simulink library "dspsigops"  (Simulink 6.0)
settings: Solver=ode45  SolverMode=SingleTasking  StartTime=0.0  StopTime=10.0  RelTol=1e-3
values from neighbouring files (symbols this model uses):
  b = tmp(end-3:end)    [aboutdspblks.m]    (also in dspcsum.m = find_system(blk,'LookUnderMasks','all', 'FollowLinks','on', ; dspfdes.m = []; dsprprim.m = b+Li)
settings Model: RequirementInfo=9  CovMetricSettings=d  ForwardingTableString=||__slOldName__||dspsigops/Integer Delay||__slNewName__||dspobslib/Integer Delay  Creator=szlotkin  LastModifiedBy=mlongfri  ExtModeAutoUpdateStatusClock=off  ProdHWDeviceType=Specified
settings DataIOCC: SignalLoggingName=logsOut
settings OptimizationCC: BooleanDataType=off
settings DebuggingCC: CheckExecutionContextPreStartOutputMsg=on  CheckExecutionContextRuntimeOutputMsg=on  SolverPrmCheckMsg=none
settings HardwareCC: ProdHWDeviceType=Specified  TargetUnknown=on
settings ModelReferenceCC: UpdateModelReferenceTargets=IfOutOfDate
settings SFSimCC: SFSimApplyToAllLibs=on  SFSimBuildMode=Incremental

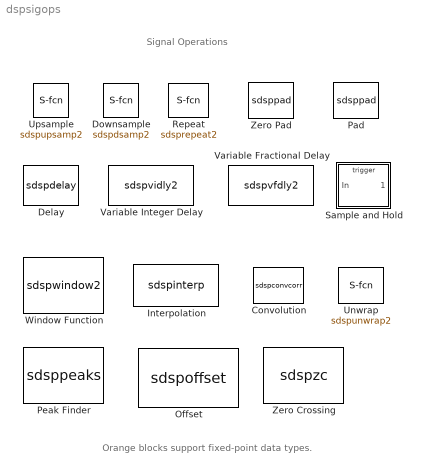
== system dspsigops ==
  note: Signal Operations
  note: Orange blocks support fixed-point data types.
  Convolution : S-Function  DialogController=dspDDGCreate  DialogControllerArgs=DataTag0  FunctionName=sdspconvcorr  Parameters=domain,0,dtInfo.prodOutputMode,dtInfo.prodOutputWordLength,dtInfo.prodOutputFracLength,dtInfo.accumMode,dtInfo.accumWordLength,dtInfo.accumFracLength,dtInfo.outputMode,dtInfo.outputWordLength,dtInfo.outputFracLength,dtInfo.roundingMode,dtInfo.overflowMode  mask(Convolution){domain=Time, additionalParams=off, allowOverrides=on, outputMode=Same as accumulator, outputWordLength=16, outputFracLength=15, accumMode=Inherit via internal rule, accumWordLength=32, accumFracLength=30, prodOutputMode=Inherit via internal rule, prodOutputWordLength=32, prodOutputFracLength=30, roundingMode=Floor, overflowMode=off, LockScale=off}
      mask prompts: domain "Computation domain:"; additionalParams "------- Show additional parameters -------"; allowOverrides "Allow overrides from DSP Fixed-Point Attributes blocks"; outputMode "Fixed-point output attributes:"; outputWordLength "Output word length:"; outputFracLength "Output fraction length:"; accumMode "Fixed-point accumulator attributes:"; accumWordLength "Accumulator word length:"; accumFracLength "Accumulator fraction length:"; prodOutputMode "Fixed-point product output attributes:"; prodOutputWordLength "Product output word length:"; prodOutputFracLength "Product output fraction length:"; roundingMode "Round integer calculations toward:"; overflowMode "Saturate on integer overflow"; LockScale "Lock scaling"
      mask help: Convolve two inputs. The block computes in the time domain or frequency domain. To minimize the number of computations, select "Fastest" in the Computation domain parameter. To minimize memory use, select "Time" in the Computation domain parameter.
      mask init:
      | dtInfo = dspblkconvcorr('init');
      settings: CopyFcn=dspfixptcopycallback
      mask Help: web(dspbhelp);
      mask StyleString: popup(Time|Frequency|Fastest),checkbox,checkbox,popup(Same as accumulator|Same as product output|Same as first input|Binary point scaling|Slope and bias scaling|User-defined),edit,edit,popup(Inherit via internal rule|Same as product output|Same as first input|Binary point scaling|Slope and bias scaling|User-defined),edit,edit,popup(Inherit via internal rule|Same as first input|Binary point scaling|Slope and bias scaling|User-defined),edit,edit,popup(Floor|Nearest),checkbox,checkbox
      mask Display: disp('CONV')
  Delay : S-Function  FunctionName=sdspdelay  Parameters=dly_unit, delay, ic_detail, dif_ic_for_ch, dif_ic_for_dly, ic, reset  mask(Delay){dly_unit=Sample, delay=1, ic_detail=off, dif_ic_for_ch=off, dif_ic_for_dly=off, ic=0, reset_popup=None}
      mask prompts: dly_unit "Delay units:"; delay "Delay (samples):"; ic_detail "--------------- Show additional parameters ---------------"; dif_ic_for_ch "Specify different initial conditions for each channel"; dif_ic_for_dly "Specify different initial conditions within a channel"; ic "Initial conditions:"; reset_popup "Reset port:"
      mask help: Delay the discrete-time input by a specified number of samples or frames. To specify the initial conditions, select the Show additional parameters check box.
      mask init:
      | if (~iscell(ic)) 
      | 	ic = double(ic);
      | end	
      | [str, ic] = dspblkdelay('init',&1,double(delay), ic);
      | dx = 0.01*length(str);
      | reset = reset_popup-1;
      | if (reset == 0)
      | 	s.i1 = 1; s.i1s = '';
      | 	s.i2 = 1; s.i2s = '';
      | else
      | 	s.i1 = 1; s.i1s = 'In';
      | 	s.i2 = 2; s.i2s = 'Rst';
      | end
      settings: CopyFcn=dspfixptcopycallback
      mask Help: web(dspbhelp);
      mask StyleString: popup(Samples|Frames),edit,checkbox,checkbox,checkbox,edit,popup(None|Rising edge|Falling edge|Either edge|Non-zero sample)
      mask CallbackString: dspblkdelay||dspblkdelay('icDetail')||||
      mask Display:
      | text(0.42-dx, 0.4, 'z'); text(0.5-dx, 0.6, str);
      | port_label('input',s.i1,s.i1s);
      | port_label('input',s.i2,s.i2s);
  Downsample : S-Function  FunctionName=sdspdsamp2  Parameters=N,phase,ic,smode,fmode  mask(Downsample){N=2, phase=0, ic=0, smode=Allow multirate, fmode=Maintain input frame size}
      mask prompts: N "Downsample factor, K:"; phase "Sample offset (0 to K-1):"; ic "Initial condition:"; smode "Sample-based mode:"; fmode "Frame-based mode:"
      mask help: Downsample by an integer factor. Optional sample offset must be an integer value in range (0, K-1).
      mask init:
      | [s,x,y] = dspblkdsamp2('icon',N, &1);
      settings: CopyFcn=dspfixptcopycallback
      mask Help: web(dspbhelp);
      mask StyleString: edit,edit,edit,popup(Allow multirate|Force single rate),popup(Maintain input frame size|Maintain input frame rate)
      mask Display:
      | plot(x,y);
      | text(.6,.4,s);
  Interpolation : S-Function  FunctionName=sdspinterp  Parameters=InterpSource,InterpPoints,InterpMode,interpFilter,InvalidMode  mask(Interpolation){InterpSource=Specify via dialog, InterpPoints=[1.1 4.8 2.67 1.6 3.2]', InterpMode=Linear, InterpL=3, InterpR=3, InterpAlpha=0.5, InvalidMode=Clip}
      mask prompts: InterpSource "Source of interpolation points:"; InterpPoints "Interpolation points:"; InterpMode "Interpolation mode:"; InterpL "Interpolation filter half-length:"; InterpR "Interpolation points per input sample:"; InterpAlpha "Normalized input bandwidth (0 to 1):"; InvalidMode "Out of range interpolation points:"
      mask help:
      | Interpolate values between real-valued input samples using linear or FIR interpolation.
      |
      | Specify which values to interpolate by providing a vector of interpolation points. An interpolation point of 1 refers to the first sample in the input.  To interpolate the value half-way between the second and third sample in the input, specify an interpolation point of 2.5.
      |
      | You can provide the vector of interpolation points in the parameter, "Interpolation points," or through the optional input port, "Pts," depending on the setting of the "Source of interpolation points" parameter.
      mask init:
      | ports = dspblkinterp('icon');
      | interpFilter = dspblkinterp('init', InterpR, InterpL, InterpAlpha);
      mask Help: web(dspbhelp)
      mask StyleString: popup(Specify via dialog|Input port),edit,popup(Linear|FIR),edit,edit,edit,popup(Clip|Clip and warn|Error)
      mask CallbackString: dspblkinterp||dspblkinterp||||
      mask Display:
      | disp('Interp')
      | port_label('input',ports.port1, ports.txt1);
      | port_label('input',ports.port2, ports.txt2);
      | port_label('output',ports.port3, ports.txt3);
  Offset : S-Function  FunctionName=sdspoffset  Parameters=mode,numDatOffPair,outWidthSpec,outWidth,actionOutRange  mask(Offset){mode=Remove beginning samples, numDatOffPair=2, outWidthSpec=Same as input, outWidth=9, actionOutRange=Clip}
      mask prompts: numDatOffPair "Number of input data-offset pairs:"; outWidthSpec "Output port length:"; outWidth "Output length:"; actionOutRange "Action for out of range offset value:"
      mask help: Truncates input vectors by removing or keeping beginning or ending values. The resulting vectors are either truncated again or zero-padded to a user-specified output length.
      mask init:
      | dspblkoffset(numDatOffPair);
      settings: CopyFcn=dspfixptcopycallback
      mask Help: web(dspbhelp);
      mask StyleString: popup(Remove beginning samples|Remove ending samples|Keep beginning samples|Keep ending samples),edit,popup(Same as input|User-defined),edit,popup(Clip|Clip and warn|Error)
      mask CallbackString: ||dspblkoffset;||
      mask Display: port_label('input',1, 'In1'); port_label('output',1, 'Out1'); port_label('input',2, 'O1'); port_label('input',3, 'In2'); port_label('output',2, 'Out2'); port_label('input',4, 'O2'); disp('Offset');
  Pad : S-Function  FunctionName=sdsppad  Parameters=padSigAt, padAlong, numOutRows, numOutCols, padVal, trunc_flag, padNumOutRowsSpecMethod, padNumOutColsSpecMethod  mask(Pad){padVal=1, padSigAt=End, padAlong=Columns, padNumOutRowsSpecMethod=User-specified, numOutRows=1, padNumOutColsSpecMethod=User-specified, numOutCols=1, trunc_flag=None}
      mask prompts: padVal "Value:"; padSigAt "Pad signal at:"; padAlong "Pad along:"; padNumOutRowsSpecMethod "Number of output rows:"; numOutRows "Specified number of output rows:"; padNumOutColsSpecMethod "Number of output columns:"; numOutCols "Specified number of output columns:"; trunc_flag "Action when truncation occurs:"
      mask help: Append or prepend a constant value to the input along specified dimensions. Truncation will occur if the specified number of output rows and/or columns is less than the corresponding input signal dimensions.
      settings: CopyFcn=dspfixptcopycallback
      mask Help: web(dspbhelp);
      mask StyleString: edit,popup(End|Beginning),popup(Columns|Rows|Columns and rows|None),popup(User-specified|Next power of two),edit,popup(User-specified|Next power of two),edit,popup(None|Warning|Error)
      mask CallbackString: ||dspblkpad|dspblkpad||dspblkpad||
      mask Display:
      | plot(0,0,100,100,[51 44 44 51],[92 92 8 8],[73 80 80 73],[92 92 8 8],[56 68],[80 80],[56 68],[72 72],[56 68],[64 64],[56 68],[56 56],[56 68],[48 48],[56 68],[40 40],[24 24 40 36 40 36],[52 24 24 28 24 20]);
      | plot([56 68],[20 20]);
      | plot([58 66],[12 28],[58 66],[28 12]);
  Peak Finder : S-Function  DialogController=dspDDGCreate  DialogControllerArgs=DataTag1  FunctionName=sdsppeaks  Parameters=maxPeaks,polarity,NoiseDistinguish,thresh,outputIdx,outputVal,roundingMode,overflowMode  mask(Peak Finder){polarity=Maxima and Minima, outputIdx=off, outputVal=off, maxPeaks=10, NoiseDistinguish=off, thresh=0, additionalParams=off, allowOverrides=off, roundingMode=Floor, overflowMode=off}
      mask prompts: polarity "Peak types:"; outputIdx "Output peak indices"; outputVal "Output peak values"; maxPeaks "Maximum number of peaks to find:"; NoiseDistinguish "Ignore peaks within threshold of neighboring values"; thresh "Threshold"; additionalParams "-------------- Show additional parameters ---------------"; allowOverrides "Allow overrides from DSP Fixed-Point Attributes blocks"; roundingMode "Round integer calculations toward:"; overflowMode "Saturate on integer overflow"
      mask help:
      | Output the number of extrema (maxima and minima) in an input signal.
      |
      | Optionally, the block can output the extrema indices, the extrema values,
      | and a binary indicator of whether or not the extrema are maxima or minima.
      mask init:
      | [s, dtInfo] = dspblkpeaks('icon',outputIdx,outputVal,polarity);
      | roundingMode   = dtInfo.roundingMode;
      | overflowMode   = dtInfo.overflowMode;
      settings: CopyFcn=dspfixptcopycallback
      mask Help: web(dspbhelp)
      mask StyleString: popup(Maxima|Minima|Maxima and Minima),checkbox,checkbox,edit,checkbox,edit,checkbox,checkbox,popup(Floor|Nearest),checkbox
      mask Display:
      | disp(['Find\n',s.txt]);
      | port_label('output',s.i1,s.s1);
      | port_label('output',s.i2,s.s2);
      | port_label('output',1,'Cnt');
      | port_label('output',s.i3,s.s3);
  Repeat : S-Function  FunctionName=sdsprepeat2  Parameters=N,ic,mode  mask(Repeat){N=5, ic=0, mode=Maintain input frame size}
      mask prompts: N "Repetition count:"; ic "Initial conditions:"; mode "Frame-based mode:"
      mask help: Repeat input samples N times.
      mask init:
      | s = dspblkrepeat2('icon',N, &1);
      settings: CopyFcn=dspfixptcopycallback
      mask Help: web(dspbhelp);
      mask StyleString: edit,edit,popup(Maintain input frame size|Maintain input frame rate)
      mask Display: disp(s);
  Sample and Hold : Subsystem  TreatAsAtomicUnit=on  PropExecContextAcrossSSBoundary=on  mask(Sample and Hold){trig=Rising edge, initCond=0}
      mask prompts: trig "Trigger type:"; initCond "Initial condition:"
      mask help: Sample and hold input signal.
      mask init:
      | switch trig
      | case 1, s='rising';
      | case 2, s='falling';
      | case 3, s='either';
      | end
      | set_param([gcb '/Trigger'],'triggertype',s);
      settings: CopyFcn=dspfixptcopycallback
      mask Help: web(dspbhelp);
      mask StyleString: popup(Rising edge|Falling edge|Either edge),edit
      mask Display: disp('S/H')
  Unwrap : S-Function  FunctionName=sdspunwrap2  Parameters=tol, running  mask(Unwrap){running=off, tol=pi}
      mask prompts: running "Do not unwrap phase discontinuities between successive frames"; tol "Tolerance (radians):"
      mask help:
      | Adds or subtracts appropriate multiples of 2pi to each input element to
      | remove phase discontinuities (unwrap). Inputs should be radian phase values.
      |
      | When the parameter "Do not unwrap phase discontinuities between successive frames" is unchecked, the block unwraps each input channel by considering all phase discontinuities in the channel, including those in previous frames of the channel. (For frame-based inputs, each column is a channel;  for sample-based inputs, each element is a channel.)
      |
      | When the parameter is checked, the block unwraps by considering phase discontinuities in the current frame only; the block unwraps each column of all frame-based inputs, and unwraps each column of sample-based inputs when the inputs are not row vectors.  It unwraps each row of sample-based row vectors.
      mask Help: web(dspbhelp);
      mask Display: plot(0,0,100,100,[16 16],[92 8],[8 92],[16 16],[16 48 48 80],[64 44 76 56],[64 64 58 64 70],[60 40 46 40 46],[69 82],[30 22],[],[],[52 65],[41 33])
  Upsample : S-Function  FunctionName=sdspupsamp2  Parameters=N,phase,ic,mode  mask(Upsample){N=3, phase=0, ic=0, mode=Maintain input frame size}
      mask prompts: N "Upsample factor, L:"; phase "Sample offset (0 to L-1):"; ic "Initial condition:"; mode "Frame-based mode:"
      mask help: Upsample by inserting L-1 zeros between input samples. Optional sample offset must be an integer value in range (0, L-1).
      mask init:
      | [s,x,y] = dspblkupsamp2('icon',N, &1);
      settings: CopyFcn=dspfixptcopycallback
      mask Help: web(dspbhelp);
      mask StyleString: edit,edit,edit,popup(Maintain input frame size|Maintain input frame rate)
      mask Display:
      | plot(x,y)
      | text(.6,.4,s);
  Variable Fractional Delay : S-Function  FunctionName=sdspvfdly2  Parameters=mode,dmax,b,ic  mask(Variable Fractional Delay){mode=Linear Interpolation, dmax=100, L=4, R=10, alpha=1, ic=0}
      mask prompts: dmax "Maximum delay (samples):"; L "Interpolation filter half-length:"; R "Interpolation points per input sample:"; alpha "Normalized input bandwidth (0 to 1):"; ic "Initial conditions:"
      mask help: Delay discrete-time input by a time-varying fractional number of sample periods, as specified by the "delay" input. The FIR filter is designed using "intfilt" from the Signal Processing Toolbox.
      mask init:
      | [b,str] = dspblkvfdly2(mode,R,L,alpha);
      mask Help: web(dspbhelp);
      mask StyleString: popup(Linear Interpolation|FIR Interpolation),edit,edit,edit,edit,edit
      mask CallbackString: dspblkvfdly2;|||||
      mask Display:
      | text(0.5,0.4,'z','horiz','right')
      | text(0.5,0.6,'-f','horiz','left')
      | port_label('input',1,'In')
      | port_label('input',2,'Delay')
      | port_label('output',1,'Out')
  Variable Integer Delay : S-Function  FunctionName=sdspvidly2  Parameters=dmax,ic  mask(Variable Integer Delay){dmax=100, ic=0}
      mask prompts: dmax "Maximum delay (samples):"; ic "Initial conditions:"
      mask help: Delay discrete-time input by a time-varying integer number of sample periods specified by the "delay" input.
      settings: CopyFcn=dspfixptcopycallback
      mask Help: web(dspbhelp);
      mask Display:
      | text(0.5,0.4,'z','horiz','right')
      | text(0.5,0.6,'-i','horiz','left')
      | port_label('input',1,'In')
      | port_label('input',2,'Delay')
      | port_label('output',1,'Out')
  Window Function : S-Function  DialogController=dspDDGCreate  DialogControllerArgs=DataTag2  FunctionName=sdspwindow2  Parameters=winmode,N,sampmode,samptime, dtInfo.DataTypeIsCustomFloat,dtInfo.DataTypeIsSigned,dTypeID,dtInfo.DataTypeWordLength,dtInfo.DataTypeFracOrMantBits,fixptInfo.firstCoeffMode,fixptInfo.firstCoeffWordLength,fixptInfo.firstCoeffFracLength,fixptInfo.prodOutputMode,fixptInfo.prodOutputWordLength,fixptInfo.prodOutputFracLength,fixptInfo.outputMode,fixptInfo.outputWordLength,fixptInfo.outputFracLength,fixptInfo.roundingMode,fixptInfo.overflowMode  mask(Window Function){winmode=Apply window to input, wintype=Hamming, sampmode=Continuous, samptime=1, N=64, Rs=50, beta=10, winsamp=Symmetric, UserWindow=hamming, OptParams=off, UserParams={'symmetric'}, additionalParams=off, allowOverrides=on, dataType=double, isSigned=on, wordLen=16, udDataType=sfix(16), fracBitsMode=Best precision, numFracBits=15, firstCoeffMode=Same word length as input, firstCoeffWordLength=16, firstCoeffFracLength=15, prodOutputMode=Inherit via internal rule, prodOutputWordLength=16, prodOutputFracLength=15, outputMode=Same as product output, outputWordLength=16, outputFracLength=15, roundingMode=Floor, overflowMode=off, LockScale=off}
      mask prompts: winmode "Operation:"; wintype "Window type:"; sampmode "Sample mode:"; samptime "Sample time:"; N "Window length:"; Rs "Stopband attenuation in dB:"; winsamp "Sampling:"; UserWindow "Window function name:"; OptParams "Additional parameters for user defined window"; UserParams "Window function parameters:"; additionalParams "------- Show additional parameters --------"; allowOverrides "Allow overrides from DSP Fixed-Point Attributes blocks"; dataType "Output data type:"; isSigned "Signed"; wordLen "Word length:"; udDataType "User-defined data type  (e.g. sfix(16), float('single')):"; fracBitsMode "Set fraction length in output to:"; numFracBits "Fraction length:"; firstCoeffMode "Fixed-point window attributes:"; firstCoeffWordLength "Window word length:"; firstCoeffFracLength "Window fraction length:"; prodOutputMode "Fixed-point product output attributes:"; prodOutputWordLength "Product output word length:"; prodOutputFracLength "Product output fraction length:"; outputMode "Fixed-point output attributes:"; outputWordLength "Output word length:"; outputFracLength "Output fraction length:"; roundingMode "Round integer calculations towards:"; overflowMode "Saturate on integer overflow"; LockScale "Lock scaling"
      mask help:
      | Generate a window function and/or apply a window function to an input signal.
      |
      | For some fixed-point modes, the fraction length or slope of the window values is automatically set for you to the best possible precision given the real-world values and word length of the window values. This is equivalent to the ''Best Precision: Matrix-wise'' scaling option used in some Simulink fixed-point blocks.
      mask init:
      | [x,y,str,ports,w,dtInfo,dTypeID,fixptInfo]=dspblkwinfcn2('init');
      settings: CopyFcn=dspfixptcopycallback
      mask Help: web(dspbhelp);
      mask StyleString: popup(Apply window to input|Generate window|Generate and apply window),popup(Bartlett|Blackman|Boxcar|Chebyshev|Hamming|Hann|Hanning|Kaiser|Triang|User defined),popup(Discrete|Continuous),edit,edit,edit,edit,popup(Symmetric|Periodic),edit,checkbox,edit,checkbox,checkbox,popup(double|single|Fixed-point|User-defined|Inherit via back propagation),checkbox,edit,edit,popup(Best precision|User-defined),edit,popup(Same word length as input|Specify word length|Binary point scaling|Slope and bias scaling|User-defined),edit,edit,popup(Inherit via internal rule|Same as input|Binary point scaling|Slope and bias scaling|User-defined),edit,edit,popup(Same as product output|Same as input|Binary point scaling|Slope and bias scaling|User-defined),edit,edit,popup(Floor|Nearest),checkbox,checkbox
      mask Display:
      | plot(x,y); text(.2,.85,str);
      | port_label(ports(1).type,ports(1).port,ports(1).txt);
      | port_label(ports(2).type,ports(2).port,ports(2).txt);
      | port_label(ports(3).type,ports(3).port,ports(3).txt);
  Zero Crossing : S-Function  FunctionName=sdspzc  Parameters=1,1
      settings: CopyFcn=dspfixptcopycallback
      mask Type: Zero Crossing
      mask Description: Counts the number of zero crossings in a signal.
      mask Help: web(dspbhelp)
      mask Display:
      | disp(['Zero\nCrossing']);
      | port_label('output',1,'Cnt');
  Zero Pad : S-Function  FunctionName=sdsppad  Parameters=padSigAt, zpadAlong, numOutRows, numOutCols, 0, trunc_flag, padNumOutRowsSpecMethod, padNumOutColsSpecMethod  mask(Zero Pad){padSigAt=End, zpadAlong=Columns, padNumOutRowsSpecMethod=User-specified, numOutRows=1, padNumOutColsSpecMethod=User-specified, numOutCols=1, trunc_flag=None}
      mask prompts: padSigAt "Pad signal at:"; zpadAlong "Pad along:"; padNumOutRowsSpecMethod "Number of output rows:"; numOutRows "Specified number of output rows:"; padNumOutColsSpecMethod "Number of output columns:"; numOutCols "Specified number of output columns:"; trunc_flag "Action when truncation occurs:"
      mask help: Append or prepend zeros to the input along specified dimensions. Truncation will occur if the specified number of output rows and/or columns is less than the corresponding input signal dimensions.
      settings: CopyFcn=dspfixptcopycallback
      mask Help: web(dspbhelp);
      mask StyleString: popup(End|Beginning),popup(Columns|Rows|Columns and rows|None),popup(User-specified|Next power of two),edit,popup(User-specified|Next power of two),edit,popup(None|Warning|Error)
      mask CallbackString: |dspblkzpad2|dspblkzpad2||dspblkzpad2||
      mask Display: plot(0,0,100,100,[51 44 44 51],[92 92 8 8],[73 80 80 73],[92 92 8 8],[56 68],[80 80],[56 68],[72 72],[56 68],[64 64],[56 68],[56 56],[56 68],[48 48],[56 68],[40 40],[64 60 56 55 56 60 64 68 69 68 64],[32 32 28 22 16 12 12 16 22 28 32],[24 24 40 36 40 36],[52 24 24 28 24 20])

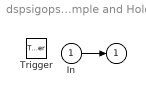
== system dspsigops/Sample and Hold ==
  In : Inport  LatchInput=off
  Trigger : TriggerPort  ZeroCross=off
  " " : Outport  InitialOutput=initCond
  wires:
  In/1 -> " "/1
